simulink model "lab12"  (R2020a)
settings: Solver=VariableStepAuto  StartTime=0.0  StopTime=10.0  RelTol=1e-3
settings Model: Creator=ILIA  LastModifiedBy=ILIA

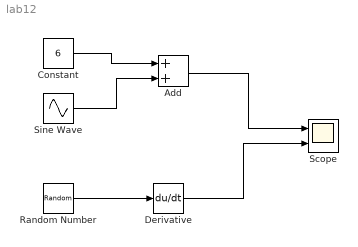
== system lab12 ==
  Add : Sum
  Constant : Constant  Value=6
  Derivative : Derivative
  Random Number : RandomNumber  SampleTime=0.1
  Scope : Scope  NumInputPorts=2
  Sine Wave : Sin  SampleTime=0
  wires:
  Constant/1 -> Add/1
  Sine Wave/1 -> Add/2
  Add/1 -> Scope/1
  Random Number/1 -> Derivative/1
  Derivative/1 -> Scope/2
